simulink library "dual_threephase_voltage_current_measure"  (R2025b)
settings: Solver=VariableStepAuto  StartTime=0.0  StopTime=10.0  RelTol=1e-3
libraries: fl_lib x18, nesl_utility x12
settings Model: Creator=ltnbda  LastModifiedBy=ltnbda

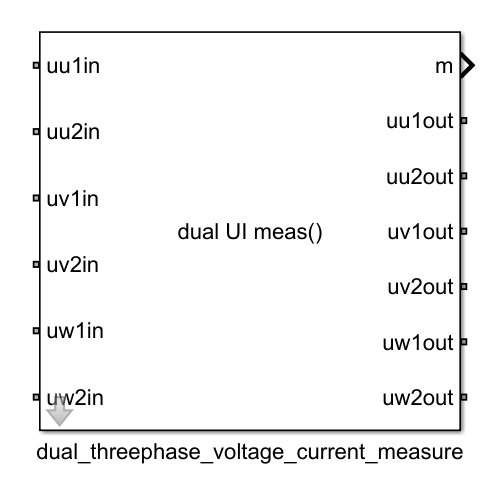
[thumbnail: Simulink's stored preview of the top-level diagram]
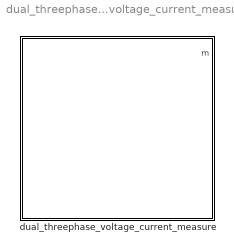
== system dual_threephase_voltage_current_measure ==
  dual_threephase_voltage_current_measure : Subsystem
      mask Display:
      | disp('dual UI meas()');
      | 
      | port_label('lconn', 1, 'uu1in');
      | port_label('lconn', 2, 'uu2in');
      | port_label('lconn', 3, 'uv1in');
      | port_label('lconn', 4, 'uv2in');
      | port_label('lconn', 5, 'uw1in');
      | port_label('lconn', 6, 'uw2in');
      | 
      | port_label('rconn', 1, 'uu1out');
      | port_label('rconn', 2, 'uu2out');
      | port_label('rconn', 3, 'uv1out');
      | port_label('rconn', 4, 'uv2out');
      | port_label('rconn', 5, 'uw1out');
      | port_label('rconn', 6, 'uw2out');
      | 
      | port_label('output', 1, 'm');

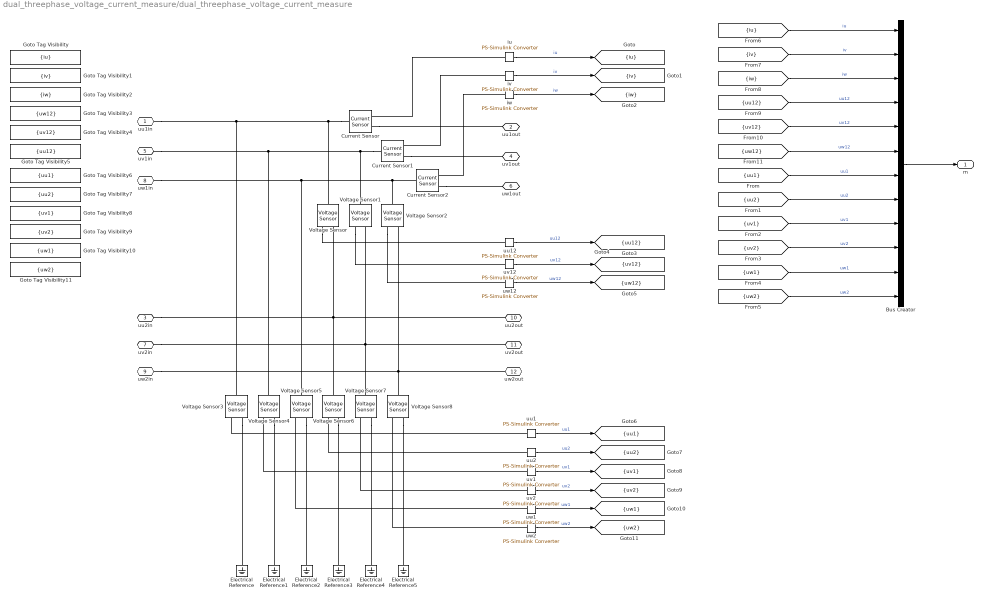
== system dual_threephase_voltage_current_measure/dual_threephase_voltage_current_measure ==
  Bus Creator : BusCreator  Inputs=12
  Current Sensor : fl_lib/Electrical/Electrical Sensors/Current Sensor
  Current Sensor1 : fl_lib/Electrical/Electrical Sensors/Current Sensor
  Current Sensor2 : fl_lib/Electrical/Electrical Sensors/Current Sensor
  Electrical Reference{,1..5} (6 alike) : fl_lib/Electrical/Electrical Elements/Electrical Reference
  Goto Tag Visibility : GotoTagVisibility  GotoTag=iu
  Goto Tag Visibility1 : GotoTagVisibility  GotoTag=iv
  Goto Tag Visibility10 : GotoTagVisibility  GotoTag=uw1
  Goto Tag Visibility11 : GotoTagVisibility  GotoTag=uw2
  Goto Tag Visibility2 : GotoTagVisibility  GotoTag=iw
  Goto Tag Visibility3 : GotoTagVisibility  GotoTag=uw12
  Goto Tag Visibility4 : GotoTagVisibility  GotoTag=uv12
  Goto Tag Visibility5 : GotoTagVisibility  GotoTag=uu12
  Goto Tag Visibility6 : GotoTagVisibility  GotoTag=uu1
  Goto Tag Visibility7 : GotoTagVisibility  GotoTag=uu2
  Goto Tag Visibility8 : GotoTagVisibility  GotoTag=uv1
  Goto Tag Visibility9 : GotoTagVisibility  GotoTag=uv2
  Voltage Sensor{,1..8} (9 alike) : fl_lib/Electrical/Electrical Sensors/Voltage Sensor
  iu : nesl_utility/PS-Simulink Converter  PhysicalDomain=network_engine_domain  SubClassName=ps_output  LeftPortType=input  RightPortType=output  PseudoPeriodic=off  Frequencies=[]  VectorFormat=1-D array  Unit=A  AffineConversion=off
  iv : nesl_utility/PS-Simulink Converter  PhysicalDomain=network_engine_domain  SubClassName=ps_output  LeftPortType=input  RightPortType=output  PseudoPeriodic=off  Frequencies=[]  VectorFormat=1-D array  Unit=A  AffineConversion=off
  iw : nesl_utility/PS-Simulink Converter  PhysicalDomain=network_engine_domain  SubClassName=ps_output  LeftPortType=input  RightPortType=output  PseudoPeriodic=off  Frequencies=[]  VectorFormat=1-D array  Unit=A  AffineConversion=off
  uu1 : nesl_utility/PS-Simulink Converter  PhysicalDomain=network_engine_domain  SubClassName=ps_output  LeftPortType=input  RightPortType=output  PseudoPeriodic=off  Frequencies=[]  VectorFormat=1-D array  Unit=V  AffineConversion=off
  uu12 : nesl_utility/PS-Simulink Converter  PhysicalDomain=network_engine_domain  SubClassName=ps_output  LeftPortType=input  RightPortType=output  PseudoPeriodic=off  Frequencies=[]  VectorFormat=1-D array  Unit=V  AffineConversion=off
  uu2 : nesl_utility/PS-Simulink Converter  PhysicalDomain=network_engine_domain  SubClassName=ps_output  LeftPortType=input  RightPortType=output  PseudoPeriodic=off  Frequencies=[]  VectorFormat=1-D array  Unit=V  AffineConversion=off
  uv1 : nesl_utility/PS-Simulink Converter  PhysicalDomain=network_engine_domain  SubClassName=ps_output  LeftPortType=input  RightPortType=output  PseudoPeriodic=off  Frequencies=[]  VectorFormat=1-D array  Unit=V  AffineConversion=off
  uv12 : nesl_utility/PS-Simulink Converter  PhysicalDomain=network_engine_domain  SubClassName=ps_output  LeftPortType=input  RightPortType=output  PseudoPeriodic=off  Frequencies=[]  VectorFormat=1-D array  Unit=V  AffineConversion=off
  uv2 : nesl_utility/PS-Simulink Converter  PhysicalDomain=network_engine_domain  SubClassName=ps_output  LeftPortType=input  RightPortType=output  PseudoPeriodic=off  Frequencies=[]  VectorFormat=1-D array  Unit=V  AffineConversion=off
  uw1 : nesl_utility/PS-Simulink Converter  PhysicalDomain=network_engine_domain  SubClassName=ps_output  LeftPortType=input  RightPortType=output  PseudoPeriodic=off  Frequencies=[]  VectorFormat=1-D array  Unit=V  AffineConversion=off
  uw12 : nesl_utility/PS-Simulink Converter  PhysicalDomain=network_engine_domain  SubClassName=ps_output  LeftPortType=input  RightPortType=output  PseudoPeriodic=off  Frequencies=[]  VectorFormat=1-D array  Unit=V  AffineConversion=off
  uw2 : nesl_utility/PS-Simulink Converter  PhysicalDomain=network_engine_domain  SubClassName=ps_output  LeftPortType=input  RightPortType=output  PseudoPeriodic=off  Frequencies=[]  VectorFormat=1-D array  Unit=V  AffineConversion=off
  uu1in : PMIOPort  Side=Left
  uu1out : PMIOPort  Port=2  Side=Right
  uu2in : PMIOPort  Port=3  Side=Left
  uv1out : PMIOPort  Port=4  Side=Right
  uv1in : PMIOPort  Port=5  Side=Left
  uw1out : PMIOPort  Port=6  Side=Right
  uv2in : PMIOPort  Port=7  Side=Left
  uw1in : PMIOPort  Port=8  Side=Left
  uw2in : PMIOPort  Port=9  Side=Left
  uu2out : PMIOPort  Port=10  Side=Right
  uv2out : PMIOPort  Port=11  Side=Right
  uw2out : PMIOPort  Port=12  Side=Right
  m : Outport
  tag scope: iu=scoped, iv=scoped, iw=scoped, uu12=scoped, uu1=scoped, uu2=scoped, uv12=scoped, uv1=scoped, uv2=scoped, uw12=scoped, uw1=scoped, uw2=scoped
  wires:
  iu/1 -> [iu]  "iu"
  iv/1 -> [iv]  "iv"
  iw/1 -> [iw]  "iw"
  uv12/1 -> [uv12]  "uv12"
  uu12/1 -> [uu12]  "uu12"
  uw12/1 -> [uw12]  "uw12"
  uu1/1 -> [uu1]  "uu1"
  uu2/1 -> [uu2]  "uu2"
  uv2/1 -> [uv2]  "uv2"
  uv1/1 -> [uv1]  "uv1"
  uw2/1 -> [uw2]  "uw2"
  uw1/1 -> [uw1]  "uw1"
  [iu] -> Bus Creator/1  "iu"
  [iv] -> Bus Creator/2  "iv"
  [iw] -> Bus Creator/3  "iw"
  [uu12] -> Bus Creator/4  "uu12"
  [uv12] -> Bus Creator/5  "uv12"
  [uw12] -> Bus Creator/6  "uw12"
  [uu1] -> Bus Creator/7  "uu1"
  [uu2] -> Bus Creator/8  "uu2"
  [uv1] -> Bus Creator/9  "uv1"
  [uv2] -> Bus Creator/10  "uv2"
  [uw1] -> Bus Creator/11  "uw1"
  [uw2] -> Bus Creator/12  "uw2"
  Bus Creator/1 -> m/1
  connections:
  Current Sensor1/LConn1 -- Voltage Sensor1/LConn1 -- uv1in/RConn1 -- Voltage Sensor4/LConn1
  Voltage Sensor/RConn1 -- uu12/LConn1
  Current Sensor/RConn2 -- uu1out/RConn1
  Voltage Sensor1/RConn1 -- uv12/LConn1
  Current Sensor2/LConn1 -- Voltage Sensor2/LConn1 -- uw1in/RConn1 -- Voltage Sensor5/LConn1
  Current Sensor/LConn1 -- Voltage Sensor/LConn1 -- Voltage Sensor3/LConn1 -- uu1in/RConn1
  Current Sensor1/RConn2 -- uv1out/RConn1
  Voltage Sensor2/RConn1 -- uw12/LConn1
  iv/LConn1 -- Current Sensor1/RConn1
  iu/LConn1 -- Current Sensor/RConn1
  iw/LConn1 -- Current Sensor2/RConn1
  Current Sensor2/RConn2 -- uw1out/RConn1
  Voltage Sensor/RConn2 -- uu2out/RConn1 -- uu2in/RConn1 -- Voltage Sensor6/LConn1
  Voltage Sensor1/RConn2 -- uv2in/RConn1 -- uv2out/RConn1 -- Voltage Sensor7/LConn1
  uw2in/RConn1 -- uw2out/RConn1 -- Voltage Sensor2/RConn2 -- Voltage Sensor8/LConn1
  Voltage Sensor3/RConn2 -- Electrical Reference/LConn1
  Voltage Sensor4/RConn2 -- Electrical Reference1/LConn1
  Voltage Sensor5/RConn2 -- Electrical Reference2/LConn1
  Voltage Sensor6/RConn2 -- Electrical Reference3/LConn1
  Voltage Sensor7/RConn2 -- Electrical Reference4/LConn1
  Voltage Sensor8/RConn2 -- Electrical Reference5/LConn1
  uu1/LConn1 -- Voltage Sensor3/RConn1
  uu2/LConn1 -- Voltage Sensor6/RConn1
  uv1/LConn1 -- Voltage Sensor4/RConn1
  uv2/LConn1 -- Voltage Sensor7/RConn1
  uw1/LConn1 -- Voltage Sensor5/RConn1
  uw2/LConn1 -- Voltage Sensor8/RConn1
